simulink subsystem "lqr_controller"  (R2025b)
settings: Solver=VariableStepAuto  StartTime=0.0  StopTime=10.0  RelTol=1e-3
undefined symbols (not defined in the file or in its folder): dt_data, FT_list_ref, K
settings Model: DefaultTestHarness=lqr_controller_Harness1  Creator=kjhaydon  LastModifiedBy=kjhaydon

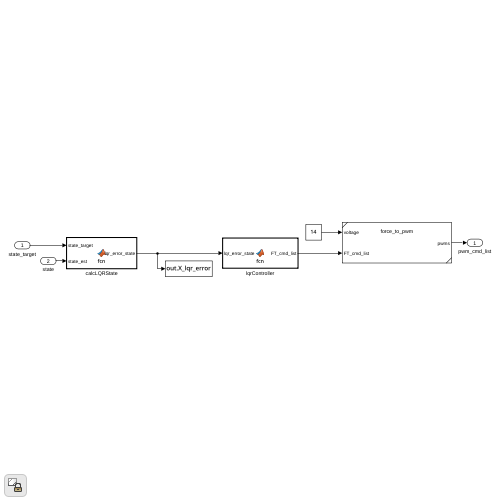
[thumbnail: Simulink's stored preview of the top-level diagram]
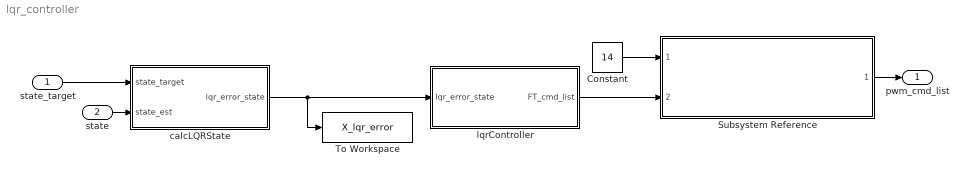
== system lqr_controller ==
  state_target : Inport
  state : Inport  Port=2
  Constant : Constant  Value=14
  Subsystem Reference : Subsystem  ReferencedSubsystem=force_to_pwm
  To Workspace : ToWorkspace  VariableName=X_lqr_error  SaveFormat=Timeseries  SampleTime=dt_data
  calcLQRState : MATLAB Function  TreatAsAtomicUnit=on
  lqrController : MATLAB Function  TreatAsAtomicUnit=on
  pwm_cmd_list : Outport
  wires:
  state_target/1 -> calcLQRState/1(state_target)
  state/1 -> calcLQRState/2(state_est)
  calcLQRState/1(lqr_error_state) -> To Workspace/1, lqrController/1(lqr_error_state)
  Subsystem Reference/1 -> pwm_cmd_list/1
  Constant/1 -> Subsystem Reference/1
  lqrController/1(FT_cmd_list) -> Subsystem Reference/2

== matlab function lqr_controller/calcLQRState ==
  data: state_target input; lqr_error_state output; state_est input
function lqr_error_state = fcn(state_target, state_est)

lqr_error_state = calcLQRState(state_target, state_est);

%angle_error = 2*qv_error

== matlab function lqr_controller/lqrController ==
  data: FT_list_ref parameter; K parameter; FT_cmd_list output; lqr_error_state input
function FT_cmd_list = fcn(FT_list_ref, K, lqr_error_state)

FT_cmd_list = lqrController(lqr_error_state, FT_list_ref, K);
